simulink model "convert_elite_individual_to_fi"  (R2024a)
settings: Solver=VariableStepAuto  StartTime=0.0  StopTime=1  RelTol=1e-3
values from neighbouring files (symbols this model uses):
  Ts = 1/Fs    (= 7.50007500075e-06)    [new_generation_coeff.m]    (also in simon_test.m; simple_fft_test.m = 1/F; testPSD_c2d.m; testPSD_simulink.m)
libraries: hdlsllib x25
settings Model: Creator=Simon  LastModifiedBy=Simon

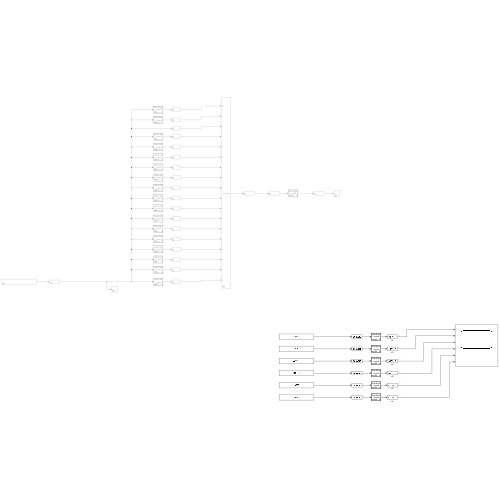
[thumbnail: Simulink's stored preview of the top-level diagram]
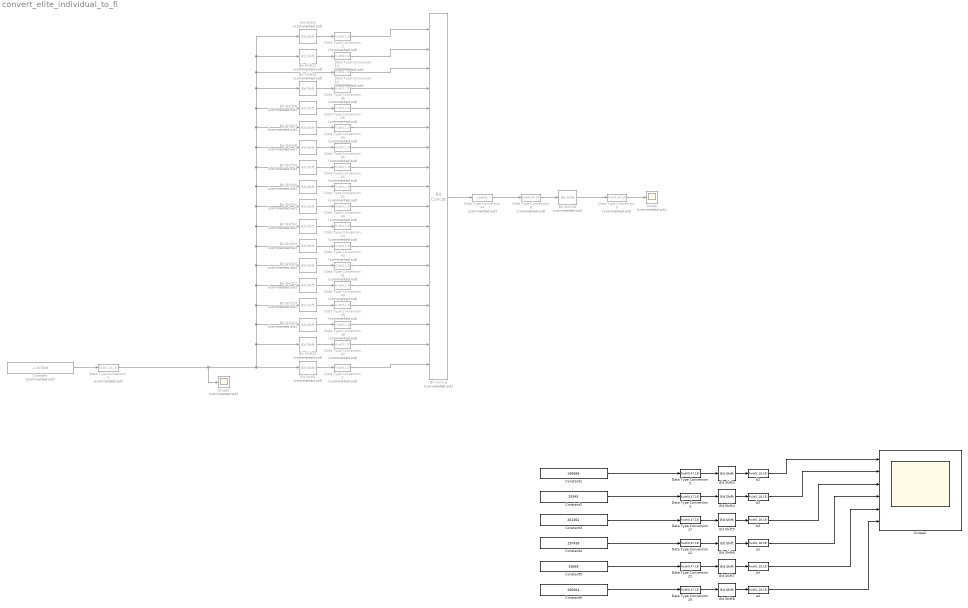
== system convert_elite_individual_to_fi ==
  Bit Concat : hdlsllib/Logic and Bit Operations/Bit Concat  Commented=on  numInputs=18
  Bit Shift1 : hdlsllib/Logic and Bit Operations/Bit Shift  Commented=on  mode=Shift Left Logical  N=15
  Bit Shift18 : hdlsllib/Logic and Bit Operations/Bit Shift  Commented=on  mode=Shift Right Logical  N=15
  Bit Shift19 : hdlsllib/Logic and Bit Operations/Bit Shift  Commented=on  mode=Shift Left Logical  N=1
  Bit Shift2 : hdlsllib/Logic and Bit Operations/Bit Shift  Commented=on  mode=Shift Right Logical  N=2
  Bit Shift20 : hdlsllib/Logic and Bit Operations/Bit Shift  Commented=on  mode=Shift Left Logical  N=10
  Bit Shift21 : hdlsllib/Logic and Bit Operations/Bit Shift  Commented=on  mode=Shift Right Logical  N=1
  Bit Shift22 : hdlsllib/Logic and Bit Operations/Bit Shift  Commented=on  mode=Shift Left Logical  N=11
  Bit Shift23 : hdlsllib/Logic and Bit Operations/Bit Shift  Commented=on  mode=Shift Left Logical  N=12
  Bit Shift24 : hdlsllib/Logic and Bit Operations/Bit Shift  Commented=on  mode=Shift Left Logical  N=13
  Bit Shift25 : hdlsllib/Logic and Bit Operations/Bit Shift  Commented=on  mode=Shift Left Logical  N=14
  Bit Shift26 : hdlsllib/Logic and Bit Operations/Bit Shift  Commented=on  mode=Shift Left Logical  N=2
  Bit Shift27 : hdlsllib/Logic and Bit Operations/Bit Shift  Commented=on  mode=Shift Left Logical  N=3
  Bit Shift28 : hdlsllib/Logic and Bit Operations/Bit Shift  Commented=on  mode=Shift Left Logical  N=4
  Bit Shift29 : hdlsllib/Logic and Bit Operations/Bit Shift  Commented=on  mode=Shift Left Logical  N=5
  Bit Shift{3..8} (6 alike) : hdlsllib/Logic and Bit Operations/Bit Shift  mode=Shift Right Logical  N=15
  Bit Shift30 : hdlsllib/Logic and Bit Operations/Bit Shift  Commented=on  mode=Shift Left Logical  N=6
  Bit Shift31 : hdlsllib/Logic and Bit Operations/Bit Shift  Commented=on  mode=Shift Left Logical  N=7
  Bit Shift32 : hdlsllib/Logic and Bit Operations/Bit Shift  Commented=on  mode=Shift Left Logical  N=8
  Bit Shift33 : hdlsllib/Logic and Bit Operations/Bit Shift  Commented=on  mode=Shift Left Logical  N=9
  Constant : Constant  Commented=on  Value=-1.457838  SampleTime=Ts
  Constant1 : Constant  Value=196684  OutDataTypeStr=uint32  SampleTime=0.1
  Constant2 : Constant  Value=33545  OutDataTypeStr=uint32  SampleTime=0.1
  Constant3 : Constant  Value=261361  OutDataTypeStr=uint32  SampleTime=0.1
  Constant4 : Constant  Value=197439  OutDataTypeStr=uint32  SampleTime=0.1
  Constant5 : Constant  Value=33669  OutDataTypeStr=uint32  SampleTime=0.1
  Constant6 : Constant  Value=260954  OutDataTypeStr=uint32  SampleTime=0.1
  Data Type Conversion{1..2,12..16,26,34..43} (18 alike) : DataTypeConversion  Commented=on  OutDataTypeStr=fixdt(0,1,0)  SaturateOnIntegerOverflow=off  RndMeth=Floor
  Data Type Conversion{3,5,17,20..22} (6 alike) : DataTypeConversion  OutDataTypeStr=fixdt(0,47,15)  SaturateOnIntegerOverflow=off  RndMeth=Floor
  Data Type Conversion4 : DataTypeConversion  Commented=on  OutDataTypeStr=fixdt(1,18,15)  SaturateOnIntegerOverflow=off  RndMeth=Floor
  Data Type Conversion44 : DataTypeConversion  Commented=on  OutDataTypeStr=uint32  SaturateOnIntegerOverflow=off  RndMeth=Floor
  Data Type Conversion8 : DataTypeConversion  Commented=on  OutDataTypeStr=fixdt(0,60,15)  SaturateOnIntegerOverflow=off  RndMeth=Floor
  Data Type Conversion9 : DataTypeConversion  Commented=on  OutDataTypeStr=fixdt(1,18,15)  SaturateOnIntegerOverflow=off  RndMeth=Floor
  Scope : Scope  Commented=on
  Scope1 : Scope  Commented=on
  Scope2 : Scope  NumInputPorts=6
  a2 : DataTypeConversion  OutDataTypeStr=fixdt(1,18,15)  SaturateOnIntegerOverflow=off  RndMeth=Floor
  a3 : DataTypeConversion  OutDataTypeStr=fixdt(1,18,15)  SaturateOnIntegerOverflow=off  RndMeth=Floor
  a4 : DataTypeConversion  OutDataTypeStr=fixdt(1,18,15)  SaturateOnIntegerOverflow=off  RndMeth=Floor
  b2 : DataTypeConversion  OutDataTypeStr=fixdt(1,18,15)  SaturateOnIntegerOverflow=off  RndMeth=Floor
  b3 : DataTypeConversion  OutDataTypeStr=fixdt(1,18,15)  SaturateOnIntegerOverflow=off  RndMeth=Floor
  b4 : DataTypeConversion  OutDataTypeStr=fixdt(1,18,15)  SaturateOnIntegerOverflow=off  RndMeth=Floor
  wires:
  Constant/1 -> Data Type Conversion4/1
  Data Type Conversion38/1 -> Bit Concat/16
  Data Type Conversion37/1 -> Bit Concat/17
  Bit Shift33/1 -> Data Type Conversion42/1
  Bit Shift23/1 -> Data Type Conversion39/1
  Bit Shift25/1 -> Data Type Conversion37/1
  Data Type Conversion41/1 -> Bit Concat/13
  Data Type Conversion43/1 -> Bit Concat/10
  Bit Shift30/1 -> Data Type Conversion15/1
  Data Type Conversion16/1 -> Bit Concat/8
  Data Type Conversion35/1 -> Bit Concat/5
  Bit Shift29/1 -> Data Type Conversion16/1
  Data Type Conversion36/1 -> Bit Concat/4
  Bit Shift1/1 -> Data Type Conversion1/1
  Bit Shift24/1 -> Data Type Conversion38/1
  Bit Shift19/1 -> Data Type Conversion36/1
  Data Type Conversion42/1 -> Bit Concat/12
  Bit Shift28/1 -> Data Type Conversion26/1
  Data Type Conversion34/1 -> Bit Concat/6
  Bit Shift21/1 -> Data Type Conversion13/1
  Data Type Conversion26/1 -> Bit Concat/7
  Bit Shift26/1 -> Data Type Conversion35/1
  Data Type Conversion1/1 -> Bit Concat/18
  Data Type Conversion13/1 -> Bit Concat/2
  Bit Shift22/1 -> Data Type Conversion40/1
  Bit Shift27/1 -> Data Type Conversion34/1
  Data Type Conversion12/1 -> Bit Concat/3
  Data Type Conversion15/1 -> Bit Concat/9
  Bit Shift2/1 -> Data Type Conversion2/1
  Data Type Conversion44/1 -> Data Type Conversion8/1
  Data Type Conversion40/1 -> Bit Concat/14
  Bit Shift32/1 -> Data Type Conversion14/1
  Data Type Conversion14/1 -> Bit Concat/11
  Bit Shift20/1 -> Data Type Conversion41/1
  Bit Shift31/1 -> Data Type Conversion43/1
  Bit Concat/1 -> Data Type Conversion44/1
  Data Type Conversion39/1 -> Bit Concat/15
  Data Type Conversion4/1 -> Scope1/1, Bit Shift25/1, Bit Shift24/1, Bit Shift23/1, Bit Shift22/1, Bit Shift20/1, Bit Shift33/1, Bit Shift32/1, Bit Shift31/1, Bit Shift30/1, Bit Shift29/1, Bit Shift28/1, Bit Shift27/1, Bit Shift26/1, Bit Shift19/1, Data Type Conversion12/1, Bit Shift2/1, Bit Shift21/1, Bit Shift1/1
  Data Type Conversion8/1 -> Bit Shift18/1
  Bit Shift18/1 -> Data Type Conversion9/1
  Data Type Conversion9/1 -> Scope/1
  Data Type Conversion2/1 -> Bit Concat/1
  b2/1 -> Scope2/1
  Bit Shift3/1 -> b2/1
  Data Type Conversion5/1 -> Bit Shift3/1
  Constant1/1 -> Data Type Conversion5/1
  Constant2/1 -> Data Type Conversion3/1
  Data Type Conversion3/1 -> Bit Shift4/1
  Bit Shift4/1 -> b3/1
  b3/1 -> Scope2/2
  b4/1 -> Scope2/3
  Bit Shift5/1 -> b4/1
  Data Type Conversion17/1 -> Bit Shift5/1
  Constant3/1 -> Data Type Conversion17/1
  Constant6/1 -> Data Type Conversion20/1
  Data Type Conversion20/1 -> Bit Shift8/1
  Bit Shift8/1 -> a4/1
  a4/1 -> Scope2/6
  a3/1 -> Scope2/5
  Bit Shift7/1 -> a3/1
  Data Type Conversion21/1 -> Bit Shift7/1
  Constant5/1 -> Data Type Conversion21/1
  Constant4/1 -> Data Type Conversion22/1
  Data Type Conversion22/1 -> Bit Shift6/1
  Bit Shift6/1 -> a2/1
  a2/1 -> Scope2/4
